simulink library "periodicCtrlExpAllocateStateMachine"  (R2020a)
settings: Solver=VariableStepAuto  StartTime=0.0  StopTime=10.0  RelTol=1e-3
undefined symbols (not defined in the file or in its folder): fltCtrl, initializeBussesFromBlock, vhcl
libraries: dspsigops x3, simulink x2, eulAng2RotMat_ul x1, periodicCtrlExpStateMachine x1, pathFollowingController_cl x1, $bdroot x1, ctrlAllocMatrixExp_cl x1
settings Model: Creator=jcreed2  LastModifiedBy=jcreed2

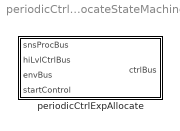
== system periodicCtrlExpAllocateStateMachine ==
  periodicCtrlExpAllocate : Subsystem  LoadFcn=initializeBussesFromBlock(gcb)  InitFcn=initializeBussesFromBlock(gcb)  mask{fltCtrl=fltCtrl}
      mask prompts: fltCtrl "Controller Model"

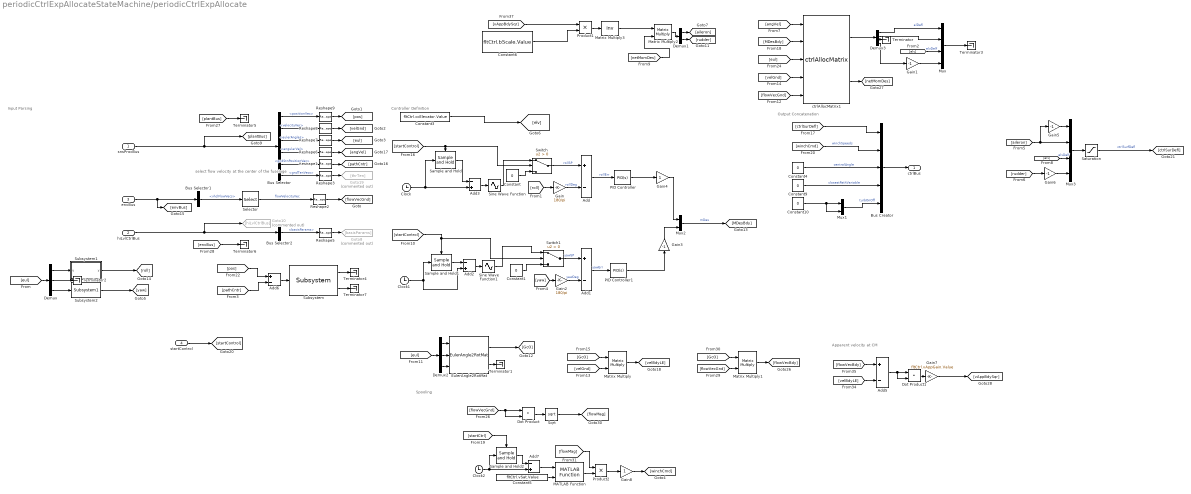
== system periodicCtrlExpAllocateStateMachine/periodicCtrlExpAllocate ==
  note: Spooling
  note: Controller Definition
  note: select flow velocity at the center of the fuselage
  note: Input Parsing
  note: Output Concatenation
  note: Apparent velocity at CM
  snsProcBus : Inport  OutDataTypeStr=Bus: sensorsProcessingBus
  hiLvlCtrlBus : Inport  Port=2  OutDataTypeStr=Bus: hiLvlCtrlBus
  envBus : Inport  Port=3  OutDataTypeStr=Bus: envBus
  startControl : Inport  Port=4
  Add{,1,5..6} (4 alike) : Sum  Inputs=+-
  Add2 : Sum  Inputs=-+
  Add3 : Sum  Inputs=-+
  Add7 : Sum  Inputs=-+
  Bus Creator : BusCreator  Inputs=5  OutDataTypeStr=Bus: fltCtrlBus
      settings: InheritFromInputs=off
  Bus Selector : BusSelector  OutputSignals=positionVec,velocityVec,eulerAngles,angularVel,gndStnPositionVec,gndTenVecs
  Bus Selector1 : BusSelector  OutputSignals=vhclFlowVecs
  Bus Selector2 : BusSelector  OutputSignals=basisParams
  Clock : Clock
  Clock1 : Clock
  Clock2 : Clock
  Constant{,1,4,9..10} (5 alike) : Constant  Value=0
  Constant3 : Constant  Value=fltCtrl.ccElevator.Value
  Constant5 : Constant  Value=fltCtrl.vSat.Value
  Constant6 : Constant  Value=fltCtrl.bScale.Value
  Demux : Demux  Outputs=3
  Demux1 : Demux  Outputs=2
  Demux2 : Demux  Outputs=3
  Demux3 : Demux
  Dot Product : DotProduct  InputSameDT=on  OutDataTypeStr=Inherit: Inherit via internal rule
  Dot Product1 : DotProduct  InputSameDT=on  OutDataTypeStr=Inherit: Inherit via internal rule
  EulerAngle2RotMat : eulAng2RotMat_ul/EulerAngle2RotMat  SystemSampleTime=-1  Latency=0  AutoFrameSizeCalculation=off
  Gain : Gain  Gain=180/pi
  Gain{1,3,5..6} (4 alike) : Gain  Gain=-1
  Gain2 : Gain  Gain=180/pi
  Gain4 : Gain
  Gain7 : Gain  Gain=fltCtrl.vAppGain.Value
  Gain8 : Gain
  Goto10 : Goto  Commented=on  GotoTag=hiLvlCtrlBus
  Goto19 : Goto  Commented=on  GotoTag=thrTen
  Goto8 : Goto  Commented=on  GotoTag=basisParams
  MATLAB Function : periodicCtrlExpStateMachine/periodicCtrlExpStateMachine/MATLAB Function  SystemSampleTime=-1  Latency=0  AutoFrameSizeCalculation=off
  Matrix Multiply : Product  Multiplication=Matrix(*)
  Matrix Multiply1 : Product  Multiplication=Matrix(*)
  Matrix Multiply2 : Product  Multiplication=Matrix(*)
  Matrix Multiply3 : Product  Inputs=/  Multiplication=Matrix(*)
  Mux : Mux
  Mux1 : Mux  Inputs=2
  Mux2 : Mux  Inputs=2
  Mux3 : Mux
  PID Controller : simulink/Continuous/PID Controller  Controller=PID  Form=Parallel  TimeDomain=Continuous-time  UseExternalTs=off  SampleTime=-1  IntegratorMethod=Forward Euler  FilterMethod=Forward Euler  ControllerParametersSource=internal  P=fltCtrl.rollCtrl.kp.Value  I=0  D=fltCtrl.rollCtrl.kd.Value  UseFilter=on  N=fltCtrl.rollCtrl.tau.Value  TunerSelectOption=Transfer Function Based (PID Tuner App)  InitialConditionSource=internal  InitialConditionForIntegrator=0  InitialConditionForFilter=0  DifferentiatorICPrevScaledInput=0  ExternalReset=none  TrackingMode=off  Kt=1  LimitOutput=off  UpperSaturationLimit=inf  LowerSaturationLimit=-inf  LinearizeAsGain=on  AntiWindupMode=none  Kb=1  POutMin=[]  POutMax=[]  IOutMin=[]  IOutMax=[]  DOutMin=[]  DOutMax=[]  NOutMin=[]  NOutMax=[]  SumOutMin=[]  SumOutMax=[]  SaturationOutMin=[]  SaturationOutMax=[]  PParamMin=[]  PParamMax=[]  IParamMin=[]  IParamMax=[]  DParamMin=[]  DParamMax=[]  NParamMin=[]  NParamMax=[]  KbParamMin=[]  KbParamMax=[]  KtParamMin=[]  KtParamMax=[]  KbOutMin=[]  KbOutMax=[]  KtOutMin=[]  KtOutMax=[]  IntegratorOutMin=[]  IntegratorOutMax=[]  FilterOutMin=[]  FilterOutMax=[]  SumI1OutMin=[]  SumI1OutMax=[]  SumI2OutMin=[]  SumI2OutMax=[]  SumI3OutMin=[]  SumI3OutMax=[]  SumI4OutMin=[]  SumI4OutMax=[]  SumDOutMin=[]  SumDOutMax=[]  DifferentiatorOutMin=[]  DifferentiatorOutMax=[]  FilterDiffOutCoefMin=[]  FilterDiffOutCoefMax=[]  ReciprocalOutMin=[]  ReciprocalOutMax=[]  SumDenOutMin=[]  SumDenOutMax=[]  SumNumOutMin=[]  SumNumOutMax=[]  DivideOutMin=[]  DivideOutMax=[]  UdiffTsProdOutMin=[]  UdiffTsProdOutMax=[]  NTsProdOutMin=[]  NTsProdOutMax=[]  UintegralTsProdOutMin=[]  UintegralTsProdOutMax=[]  UngainTsProdOutMin=[]  UngainTsProdOutMax=[]  IntegratorContinuousStateAttributes=''  IntegratorStateMustResolveToSignalObject=off  IntegratorRTWStateStorageClass=Auto  FilterContinuousStateAttributes=''  FilterStateMustResolveToSignalObject=off  FilterRTWStateStorageClass=Auto  ParallelPVariant=InternalParameters  IdealPVariant=Disabled  IVariant=InternalParameters  DVariant=InternalParameters  IntegratorVariant=Continuous  SatVariant=Disabled  AWVariant=Passthrough  PCopyVariant=Disabled  TRVariant=Disabled  FdbkBlocksVariant=Forward  IdealPFdbkVariant=Disabled  SatFdbkVariant=Disabled  DerivativeFilterVariant=ContFilter  NVariant=InternalParameters  NCopyVariant=Disabled  FilterICVariant=InternalICsFilter  IntegratorICVariant=InternalICs  ExternalResetVariant=Disabled  TRSumVariant=Passthrough  SumFdbkVariant=Disabled  SumVariant=Sum_PID  TsampFilterVariant=InternalTs  TsampNgainVariant=Passthrough  TsampIntegralVariant=Passthrough
  PID Controller1 : simulink/Continuous/PID Controller  Controller=PID  Form=Parallel  TimeDomain=Continuous-time  UseExternalTs=off  SampleTime=-1  IntegratorMethod=Forward Euler  FilterMethod=Forward Euler  ControllerParametersSource=internal  P=fltCtrl.yawCtrl.kp.Value  I=0  D=fltCtrl.yawCtrl.kd.Value  UseFilter=on  N=fltCtrl.yawCtrl.tau.Value  TunerSelectOption=Transfer Function Based (PID Tuner App)  InitialConditionSource=internal  InitialConditionForIntegrator=0  InitialConditionForFilter=0  DifferentiatorICPrevScaledInput=0  ExternalReset=none  TrackingMode=off  Kt=1  LimitOutput=off  UpperSaturationLimit=inf  LowerSaturationLimit=-inf  LinearizeAsGain=on  AntiWindupMode=none  Kb=1  POutMin=[]  POutMax=[]  IOutMin=[]  IOutMax=[]  DOutMin=[]  DOutMax=[]  NOutMin=[]  NOutMax=[]  SumOutMin=[]  SumOutMax=[]  SaturationOutMin=[]  SaturationOutMax=[]  PParamMin=[]  PParamMax=[]  IParamMin=[]  IParamMax=[]  DParamMin=[]  DParamMax=[]  NParamMin=[]  NParamMax=[]  KbParamMin=[]  KbParamMax=[]  KtParamMin=[]  KtParamMax=[]  KbOutMin=[]  KbOutMax=[]  KtOutMin=[]  KtOutMax=[]  IntegratorOutMin=[]  IntegratorOutMax=[]  FilterOutMin=[]  FilterOutMax=[]  SumI1OutMin=[]  SumI1OutMax=[]  SumI2OutMin=[]  SumI2OutMax=[]  SumI3OutMin=[]  SumI3OutMax=[]  SumI4OutMin=[]  SumI4OutMax=[]  SumDOutMin=[]  SumDOutMax=[]  DifferentiatorOutMin=[]  DifferentiatorOutMax=[]  FilterDiffOutCoefMin=[]  FilterDiffOutCoefMax=[]  ReciprocalOutMin=[]  ReciprocalOutMax=[]  SumDenOutMin=[]  SumDenOutMax=[]  SumNumOutMin=[]  SumNumOutMax=[]  DivideOutMin=[]  DivideOutMax=[]  UdiffTsProdOutMin=[]  UdiffTsProdOutMax=[]  NTsProdOutMin=[]  NTsProdOutMax=[]  UintegralTsProdOutMin=[]  UintegralTsProdOutMax=[]  UngainTsProdOutMin=[]  UngainTsProdOutMax=[]  IntegratorContinuousStateAttributes=''  IntegratorStateMustResolveToSignalObject=off  IntegratorRTWStateStorageClass=Auto  FilterContinuousStateAttributes=''  FilterStateMustResolveToSignalObject=off  FilterRTWStateStorageClass=Auto  ParallelPVariant=InternalParameters  IdealPVariant=Disabled  IVariant=InternalParameters  DVariant=InternalParameters  IntegratorVariant=Continuous  SatVariant=Disabled  AWVariant=Passthrough  PCopyVariant=Disabled  TRVariant=Disabled  FdbkBlocksVariant=Forward  IdealPFdbkVariant=Disabled  SatFdbkVariant=Disabled  DerivativeFilterVariant=ContFilter  NVariant=InternalParameters  NCopyVariant=Disabled  FilterICVariant=InternalICsFilter  IntegratorICVariant=InternalICs  ExternalResetVariant=Disabled  TRSumVariant=Passthrough  SumFdbkVariant=Disabled  SumVariant=Sum_PID  TsampFilterVariant=InternalTs  TsampNgainVariant=Passthrough  TsampIntegralVariant=Passthrough
  Product1 : Product
  Product2 : Product
  Reshape{1..3,5..9} (8 alike) : Reshape  OutputDimensionality=Column vector (2-D)
  Sample and Hold : dspsigops/Sample and Hold  trig=Rising edge  initCond=0  latchinput=off
  Sample and Hold1 : dspsigops/Sample and Hold  trig=Rising edge  initCond=0  latchinput=off
  Sample and Hold2 : dspsigops/Sample and Hold  trig=Rising edge  initCond=0  latchinput=off
  Saturation : Saturate  UpperLimit=30  LowerLimit=-30
  Selector : Selector  NumberOfDimensions=2  InputPortWidth=3  IndexOptions=Select all,Index vector (dialog)  Indices=[1 3],5  OutputSizes=1,1
  Sine Wave Function : Sin  TimeSource=Use external signal  Amplitude=fltCtrl.rollAmp.Value  Frequency=fltCtrl.frequency.Value  Phase=fltCtrl.rollPhase.Value  SampleTime=0
  Sine Wave Function1 : Sin  TimeSource=Use external signal  Amplitude=fltCtrl.yawAmp.Value  Frequency=fltCtrl.frequency.Value  Phase=fltCtrl.yawPhase.Value  SampleTime=0
  Sqrt : Sqrt  SaturateOnIntegerOverflow=on
  Subsystem : pathFollowingController_cl/pathFollowingController/Subsystem  SystemSampleTime=-1  Latency=0  AutoFrameSizeCalculation=off
  Subsystem1 : Subsystem
  Subsystem2 : $bdroot/periodicCtrlExpAllocate/Subsystem1  SystemSampleTime=-1  Latency=0  AutoFrameSizeCalculation=off
  Switch : Switch  Criteria=u2 > Threshold
  Switch1 : Switch  Criteria=u2 > Threshold
  Terminator{,1..7} (8 alike) : Terminator
  ctrlAllocMatrix1 : ctrlAllocMatrixExp_cl/ctrlAllocMatrix  aeroStruct=vhcl.struct('OCT.aeroSurf')  fluidDensity=fluidDensity
      link override momentComponentVector/rudderPortion/Constant17: Value=55-36
  ctrlBus : Outport  OutDataTypeStr=Bus: fltCtrlBus  VectorParamsAs1DForOutWhenUnconnected=off
  wires:
  Reshape1/1 -> [pathCntr]
  Reshape9/1 -> [pos]
  Bus Selector/5 -> Reshape1/1  "<gndStnPositionVec>"
  Bus Selector/3 -> Reshape7/1  "<eulerAngles>"
  Demux/2 -> Terminator2/1
  [envBus] -> Terminator6/1
  Reshape3/1 -> Goto19/1
  Demux3/4 -> Gain1/1
  Reshape5/1 -> Goto8/1
  envBus/1 -> [envBus], Bus Selector1/1
  Bus Creator/1 -> ctrlBus/1
  Bus Selector/1 -> Reshape9/1  "<positionVec>"
  [winchCmd] -> Bus Creator/2  "winchSpeeds"
  Bus Selector/4 -> Reshape6/1  "<angularVel>"
  Reshape6/1 -> [angVel]
  Bus Selector2/1 -> Reshape5/1  "<basisParams>"
  Bus Selector/2 -> Reshape8/1  "<velocityVec>"
  Demux3/1 -> Mux/1  "alDefl"
  Reshape2/1 -> [flowVecGnd]
  [elv] -> Mux/3  "elvDelf"
  [plantBus] -> Terminator5/1
  Reshape7/1 -> [eul]
  Selector/1 -> Reshape2/1  "flowVelocityVec"
  [eul] -> Demux/1
  Bus Selector/6 -> Reshape3/1  "<gndTenVecs>"
  Demux/1 -> Subsystem1/1(u)
  Demux/3 -> Subsystem2/1
  Reshape8/1 -> [velGnd]
  Bus Selector1/1 -> Selector/1  "<vhclFlowVecs>"
  [roll] -> Gain/1
  Add/1 -> PID Controller/1  "rollErr"
  Gain/1 -> Add/2  "rollDeg"
  Clock/1 -> Add3/2, Sample and Hold/1
  Mux/1 -> Terminator3/1
  Constant3/1 -> [elv]
  Sample and Hold/1 -> Add3/1
  Add3/1 -> Sine Wave Function/1
  Sine Wave Function/1 -> Switch/1
  [startControl] -> Switch/2, Sample and Hold/Trigger
  Constant/1 -> Switch/3
  Switch/1 -> Add/1  "rollSP"
  Constant4/1 -> Bus Creator/3  "centralAngle"
  Constant9/1 -> Bus Creator/4  "closestPathVariable"
  Constant10/1 -> Mux1/2, Mux1/1
  Mux1/1 -> Bus Creator/5  "turbOnOff"
  [startControl] -> Switch1/2, Sample and Hold1/Trigger
  Constant1/1 -> Switch1/3
  Switch1/1 -> Add1/1  "yawSP"
  Add2/1 -> Sine Wave Function1/1
  Gain2/1 -> Add1/2  "yawDeg"
  [yaw] -> Gain2/1
  Sample and Hold1/1 -> Add2/1
  Clock1/1 -> Sample and Hold1/1, Add2/2
  Add1/1 -> PID Controller1/1  "yawErr"
  snsProcBus/1 -> Bus Selector/1, [plantBus]
  hiLvlCtrlBus/1 -> Goto10/1, Bus Selector2/1
  PID Controller/1 -> Gain4/1
  PID Controller1/1 -> Gain3/1
  [ctrlSurDefl] -> Bus Creator/1
  Sine Wave Function1/1 -> Switch1/1
  [vAppBdySqr] -> Product1/1
  Product1/1 -> Matrix Multiply3/1
  Constant6/1 -> Product1/2
  Matrix Multiply3/1 -> Matrix Multiply2/1
  Mux2/1 -> [MDesBdy]  "mDes"
  Matrix Multiply2/1 -> Demux1/1
  Demux1/1 -> [aileron]
  Demux1/2 -> [rudder]
  Add5/1 -> Dot Product1/2, Dot Product1/1
  [flowVecBdy] -> Add5/1
  EulerAngle2RotMat/1 -> [GcO]
  Demux2/2 -> EulerAngle2RotMat/2
  Demux2/1 -> EulerAngle2RotMat/1
  Demux2/3 -> EulerAngle2RotMat/3
  [velGnd] -> Matrix Multiply/2
  [eul] -> Demux2/1
  Matrix Multiply1/1 -> [flowVecBdy]
  Matrix Multiply/1 -> [velBdyLE]
  [flowVecGnd] -> Matrix Multiply1/2
  [GcO] -> Matrix Multiply1/1
  [GcO] -> Matrix Multiply/1
  [velBdyLE] -> Add5/2
  EulerAngle2RotMat/2 -> Terminator1/1
  Dot Product1/1 -> Gain7/1
  Gain3/1 -> Mux2/2
  Gain4/1 -> Mux2/1
  [angVel] -> ctrlAllocMatrix1/1
  [MDesBdy] -> ctrlAllocMatrix1/2
  [eul] -> ctrlAllocMatrix1/3
  [velGnd] -> ctrlAllocMatrix1/4
  [flowVecGnd] -> ctrlAllocMatrix1/5
  ctrlAllocMatrix1/2 -> [netMomDes]
  ctrlAllocMatrix1/1 -> Demux3/1
  Demux3/2 -> Mux/2
  Demux3/3 -> Terminator/1
  Gain1/1 -> Mux/4
  Subsystem/1 -> Terminator4/1
  [pos] -> Add6/1
  Subsystem/2 -> Terminator7/1
  [pathCntr] -> Add6/2
  Add6/1 -> Subsystem/1
  Mux3/1 -> Saturation/1
  [aileron] -> Gain5/1, Mux3/2
  Gain5/1 -> Mux3/1
  [elv] -> Mux3/3  "elvDelf"
  [rudder] -> Gain6/1
  Gain6/1 -> Mux3/4
  Saturation/1 -> [ctrlSurDefl]  "ctrlSurfDefl"
  [netMomDes] -> Matrix Multiply2/2
  startControl/1 -> [startControl]
  Subsystem1/1(y) -> [roll]
  Subsystem2/1 -> [yaw]
  Gain7/1 -> [vAppBdySqr]
  Clock2/1 -> Sample and Hold2/1, Add7/2
  Dot Product/1 -> Sqrt/1
  Sqrt/1 -> [flowMag]
  Product2/1 -> Gain8/1
  [startCtrl] -> Sample and Hold2/Trigger
  [flowVecGnd] -> Dot Product/1, Dot Product/2
  [flowMag] -> Product2/1
  Gain8/1 -> [winchCmd]
  Add7/1 -> MATLAB Function/1
  MATLAB Function/1 -> Product2/2
  Constant5/1 -> MATLAB Function/2
  Sample and Hold2/1 -> Add7/1

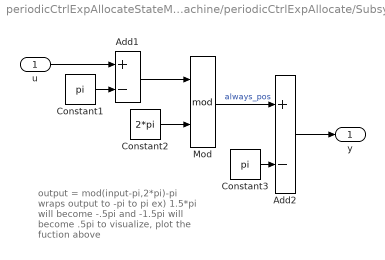
== system periodicCtrlExpAllocateStateMachine/periodicCtrlExpAllocate/Subsystem1 ==
  note: output = mod(input-pi,2*pi)-pi
      | wraps output to -pi to pi
      |
      | ex) 1.5*pi will become -.5pi
      | 	and -1.5pi will become .5pi
      |
      | to visualize, plot the fuction above
  u : Inport
  Add1 : Sum  Inputs=+-
  Add2 : Sum  Inputs=+-
  Constant1 : Constant  Value=pi
  Constant2 : Constant  Value=2*pi
  Constant3 : Constant  Value=pi
  Mod : Math  Operator=mod  SignedPower=on  SaturateOnIntegerOverflow=on
  y : Outport  VectorParamsAs1DForOutWhenUnconnected=off
  wires:
  Constant1/1 -> Add1/2
  Mod/1 -> Add2/1  "always_pos"
  Add2/1 -> y/1
  Constant2/1 -> Mod/2
  Constant3/1 -> Add2/2
  u/1 -> Add1/1
  Add1/1 -> Mod/1
